simulink model "Collision_assist_system_24_08_23_new1232020"  (R2020b)
settings: Solver=FixedStepDiscrete  StartTime=0  StopTime=100  FixedStep=0.1  RelTol=1e-3
model workspace (MAT data in the model file):
  Activate_AEB = 2
  Do_nothing = 0
  M = 3
  Match_relative_speed = 1
libraries: simulink x21
settings Model: Creator=Manohar  LastModifiedBy=Manohar
settings DebuggingCC: SFUnusedDataAndEventsDiag=none  SFUnexpectedBacktrackingDiag=none  SFInvalidInputDataAccessInChartInitDiag=none  SFNoUnconditionalDefaultTransitionDiag=none  SFUndirectedBroadcastEventsDiag=none  SFOutputUsedAsStateInMooreChartDiag=none  SFMachineParentedDataDiag=none

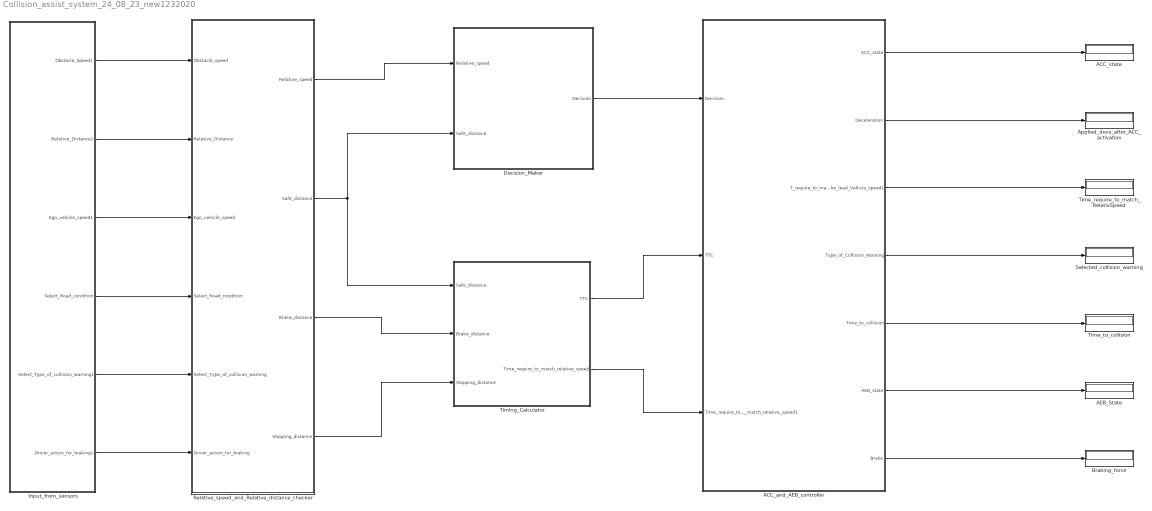
== system Collision_assist_system_24_08_23_new1232020 ==
  ACC_and_AEB_controller : Subsystem
  ACC_state : Display
  AEB_State : Display
  Applied_dece_after_ACC_activation : Display
  Braking_force : Display
  Decision_Maker : Subsystem
  Input_from_sensors : Subsystem
  Relative_speed_and_Relative_distance_checker : Subsystem
  Selected_collision_warning : Display
  Time_require_to_match_RelativSpeed : Display
  Time_to_collision : Display
  Timing_Calculator : Subsystem
  wires:
  Timing_Calculator/1(TTC) -> ACC_and_AEB_controller/2(TTC)
  ACC_and_AEB_controller/4(Type_of_Collision_Warning) -> Selected_collision_warning/1
  ACC_and_AEB_controller/5(Time_to_collision) -> Time_to_collision/1
  ACC_and_AEB_controller/6(AEB_state) -> AEB_State/1
  Relative_speed_and_Relative_distance_checker/2(Safe_distance) -> Timing_Calculator/1(Safe_distance), Decision_Maker/2(Safe_distance)
  Relative_speed_and_Relative_distance_checker/1(Relative_speed) -> Decision_Maker/1(Relative_speed)
  Relative_speed_and_Relative_distance_checker/3(Brake_distance) -> Timing_Calculator/2(Brake_distance)
  Relative_speed_and_Relative_distance_checker/4(Stopping_distance) -> Timing_Calculator/3(Stopping_distance)
  ACC_and_AEB_controller/7(Brake) -> Braking_force/1
  Decision_Maker/1(Decision) -> ACC_and_AEB_controller/1(Decision)
  Timing_Calculator/2(Time_require_to_match_relative_speed) -> ACC_and_AEB_controller/3(Time_require_to_match_relative_speed1)
  ACC_and_AEB_controller/2(Deceleration) -> Applied_dece_after_ACC_activation/1
  ACC_and_AEB_controller/1(ACC_state) -> ACC_state/1
  ACC_and_AEB_controller/3(T_require_to_match_the_lead_Vehicle_speed1) -> Time_require_to_match_RelativSpeed/1
  Input_from_sensors/1(Obstacle_Speed1) -> Relative_speed_and_Relative_distance_checker/1(Obstacle_speed)
  Input_from_sensors/2(Relative_Distance1) -> Relative_speed_and_Relative_distance_checker/2(Relative_Distance)
  Input_from_sensors/3(Ego_vehicle_speed1) -> Relative_speed_and_Relative_distance_checker/3(Ego_vehicle_speed)
  Input_from_sensors/4(Select_Road_condition) -> Relative_speed_and_Relative_distance_checker/4(Select_Road_condition)
  Input_from_sensors/5(Select_Type_of_collision_warning1) -> Relative_speed_and_Relative_distance_checker/5(Select_Type_of_collision_warning)
  Input_from_sensors/6(Driver_action_for_braking1) -> Relative_speed_and_Relative_distance_checker/6(Driver_action_for_braking)

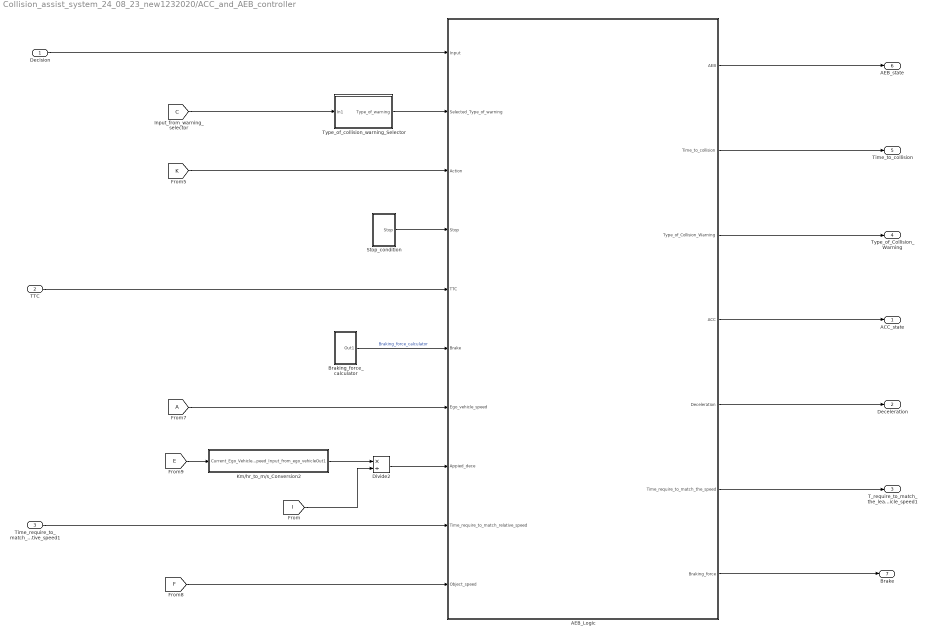
== system Collision_assist_system_24_08_23_new1232020/ACC_and_AEB_controller ==
  Decision : Inport
  TTC : Inport  Port=2
  Time_require_to_match_relative_speed1 : Inport  Port=3
  AEB_Logic : Stateflow chart  TreatAsAtomicUnit=on
      settings: PortSchema="{\"entries\":[{\"content\":{\"sides\":[{\"content\":{\"connectorIds\":[\"In5\",\"In4\",\"In3\",\"In1\",\"In2\",\"In6\",\"In7\",\"In10\",\"In8\",\"In9\"]},\"type\":\"ConnectorPlacement.EquallySpacedRectSide\",\"uuid\":\"56efa24c-13f5-4a10-8798-262846c2e7d6\"},{\"content\":{\"connectorIds\":[\"Out2\",\"Out1\",\"Out3\",\"Out5\",\"Out6\",\"Out7\",\"Out4\"],\"side\":\"RIGHT\"},\"type\":\"ConnectorPlacement.EquallySpacedRectSide\",\"uuid\":\"b772b444-91dc-49b5-b56a-5600aa3cb1ee\"},{\"content\":{\"connectorIds\":[],\"side\":\"TOP\"},\"type\":\"ConnectorPlacement.EquallySpacedRectSide\",\"uuid\":\"4494dcf3-e0bf-46dd-8a42-4684d9a2f726\"}]},\"type\":\"ConnectorPlacement.EquallySpacedConnector\",\"uuid\":\"5a6c621f-0a2a-4f9e-80e5-9478e9780666\"}],\"packageUris\":[\"http://schema.mathworks.com/mf0/Connector/R2020b\"],\"version\":\"1.0\"}"
  Braking_force_calculator : Subsystem
  Divide2 : Product  Inputs=*/
  Km/hr_to_m/s_Conversion2 : Subsystem
  Stop_condition : Subsystem
  Type_of_collision_warning_Selector : Subsystem
  ACC_state : Outport
  Deceleration : Outport  Port=2
  T_require_to_match_the_lead_Vehicle_speed1 : Outport  Port=3
  Type_of_Collision_Warning : Outport  Port=4
  Time_to_collision : Outport  Port=5
  AEB_state : Outport  Port=6
  Brake : Outport  Port=7
  wires:
  Stop_condition/1(Stop) -> AEB_Logic/1(Stop)
  [C] -> Type_of_collision_warning_Selector/1(In1)
  Type_of_collision_warning_Selector/1(Type_of_warning) -> AEB_Logic/4(Selected_Type_of_warning)
  AEB_Logic/2(AEB) -> AEB_state/1
  AEB_Logic/3(Type_of_Collision_Warning) -> Type_of_Collision_Warning/1
  TTC/1 -> AEB_Logic/2(TTC)
  [K] -> AEB_Logic/3(Action)
  AEB_Logic/4(Braking_force) -> Brake/1
  Braking_force_calculator/1(Out1) -> AEB_Logic/6(Brake)  "Braking_force_calculator"
  AEB_Logic/1(Time_to_collision) -> Time_to_collision/1
  [A] -> AEB_Logic/7(Ego_vehicle_speed)
  Divide2/1 -> AEB_Logic/10(Appied_dece)
  [E] -> Km/hr_to_m/s_Conversion2/1(Current_Ego_Vehicle_Speed_Input_from_ego_vehicle)
  Km/hr_to_m/s_Conversion2/1(Out1) -> Divide2/1
  Time_require_to_match_relative_speed1/1 -> AEB_Logic/8(Time_require_to_match_relative_speed)
  [F] -> AEB_Logic/9(Object_speed)
  AEB_Logic/6(Deceleration) -> Deceleration/1
  AEB_Logic/5(ACC) -> ACC_state/1
  AEB_Logic/7(Time_require_to_match_the_speed) -> T_require_to_match_the_lead_Vehicle_speed1/1
  Decision/1 -> AEB_Logic/5(Input)
  [I] -> Divide2/2

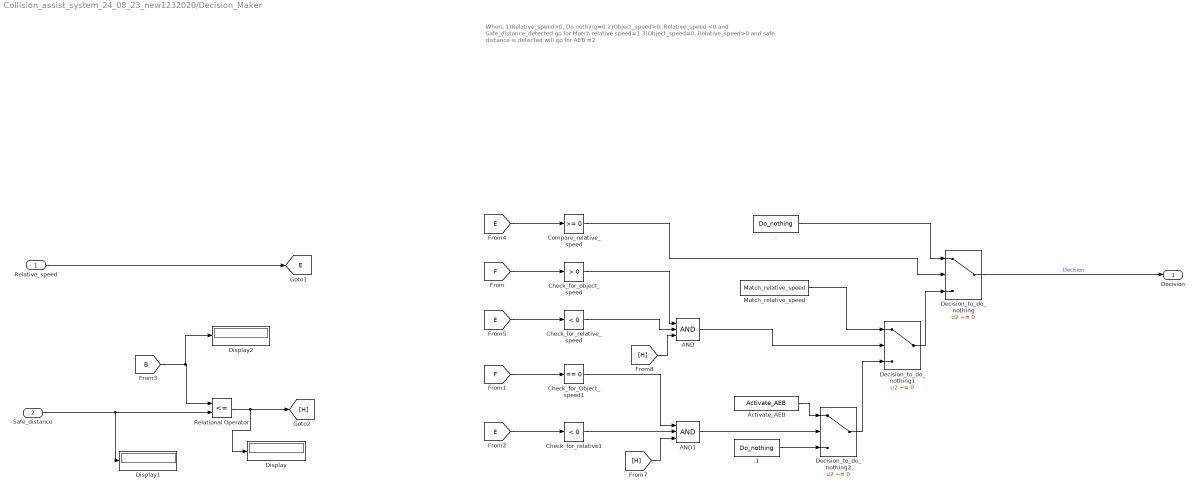
== system Collision_assist_system_24_08_23_new1232020/Decision_Maker ==
  note: When,
      | 1)Relative_speed>0, Do nothing=0
      |
      | 2)Object_speed>0, Relative_speed <0 and Safe_distance_detected go for Match relative speed=1
      |
      | 3)Object_speed=0, Relative_speed>0 and safe distance is detected will go for AEB =2
  Relative_speed : Inport
  Safe_distance : Inport  Port=2
  . : Constant  Value=Do_nothing
  .1 : Constant  Value=Do_nothing
  AND : Logic  Inputs=3  AllPortsSameDT=off  OutDataTypeStr=boolean
  AND1 : Logic  Inputs=3  AllPortsSameDT=off  OutDataTypeStr=boolean
  Activate_AEB : Constant  Value=Activate_AEB
  Check_for_Object_speed1 : simulink/Logic and Bit Operations/Compare To Constant  relop===  const=0  OutDataTypeStr=boolean
  Check_for_object_speed : simulink/Logic and Bit Operations/Compare To Constant  relop=>  const=0  OutDataTypeStr=boolean
  Check_for_relative1 : simulink/Logic and Bit Operations/Compare To Constant  relop=<  const=0  OutDataTypeStr=boolean
  Check_for_relative_speed : simulink/Logic and Bit Operations/Compare To Constant  relop=<  const=0  OutDataTypeStr=boolean
  Compare_relative_speed : simulink/Logic and Bit Operations/Compare To Constant  relop=>=  const=0  OutDataTypeStr=boolean
  Decision_to_do_nothing : Switch  Criteria=u2 ~= 0
  Decision_to_do_nothing1 : Switch  Criteria=u2 ~= 0
  Decision_to_do_nothing2 : Switch  Criteria=u2 ~= 0
  Display : Display
  Display1 : Display
  Display2 : Display
  Match_relative_speed : Constant  Value=Match_relative_speed
  Relational Operator : RelationalOperator  Operator=<=  OutDataTypeStr=boolean  RndMeth=Simplest
  Decision : Outport
  tag scope: E=global
  wires:
  [B] -> Display2/1, Relational Operator/1
  Decision_to_do_nothing1/1 -> Decision_to_do_nothing/3
  Compare_relative_speed/1 -> Decision_to_do_nothing/2
  Decision_to_do_nothing/1 -> Decision/1  "Decision"
  Match_relative_speed/1 -> Decision_to_do_nothing1/1
  ./1 -> Decision_to_do_nothing/1
  Check_for_object_speed/1 -> AND/1
  Check_for_relative_speed/1 -> AND/2
  AND/1 -> Decision_to_do_nothing1/2
  Relative_speed/1 -> [E]
  Decision_to_do_nothing2/1 -> Decision_to_do_nothing1/3
  Activate_AEB/1 -> Decision_to_do_nothing2/1
  AND1/1 -> Decision_to_do_nothing2/2
  [F] -> Check_for_object_speed/1
  [F] -> Check_for_Object_speed1/1
  [E] -> Check_for_relative1/1
  Check_for_relative1/1 -> AND1/2
  Check_for_Object_speed1/1 -> AND1/1
  Safe_distance/1 -> Display1/1, Relational Operator/2
  [E] -> Compare_relative_speed/1
  [E] -> Check_for_relative_speed/1
  Relational Operator/1 -> Display/1, [H]
  [H] -> AND1/3
  [H] -> AND/3
  .1/1 -> Decision_to_do_nothing2/3

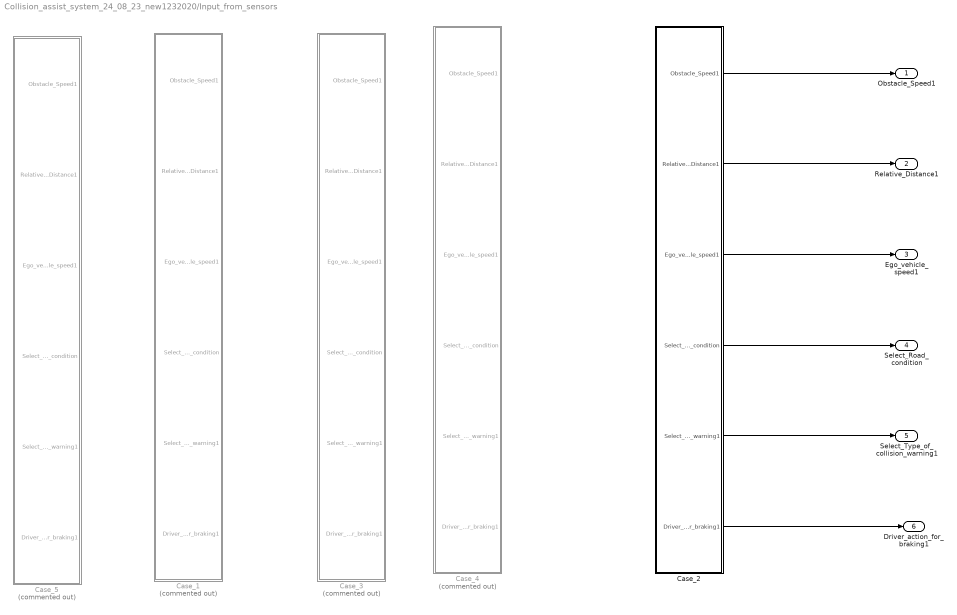
== system Collision_assist_system_24_08_23_new1232020/Input_from_sensors ==
  Case_1 : Subsystem  Commented=on
  Case_2 : Subsystem
  Case_3 : Subsystem  Commented=on
  Case_4 : Subsystem  Commented=on
  Case_5 : Subsystem  Commented=on
  Obstacle_Speed1 : Outport
  Relative_Distance1 : Outport  Port=2
  Ego_vehicle_speed1 : Outport  Port=3
  Select_Road_condition : Outport  Port=4
  Select_Type_of_collision_warning1 : Outport  Port=5
  Driver_action_for_braking1 : Outport  Port=6
  wires:
  Case_2/1(Obstacle_Speed1) -> Obstacle_Speed1/1
  Case_2/2(Relative_Distance1) -> Relative_Distance1/1
  Case_2/3(Ego_vehicle_speed1) -> Ego_vehicle_speed1/1
  Case_2/4(Select_Road_condition) -> Select_Road_condition/1
  Case_2/5(Select_Type_of_collision_warning1) -> Select_Type_of_collision_warning1/1
  Case_2/6(Driver_action_for_braking1) -> Driver_action_for_braking1/1

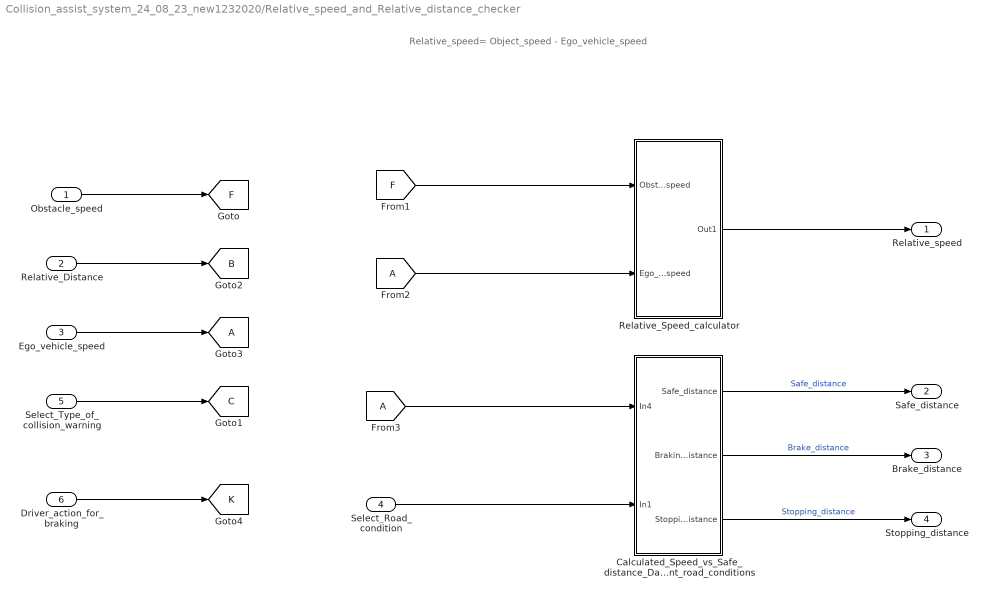
== system Collision_assist_system_24_08_23_new1232020/Relative_speed_and_Relative_distance_checker ==
  note: Relative_speed= Object_speed - Ego_vehicle_speed
  Obstacle_speed : Inport
  Relative_Distance : Inport  Port=2
  Ego_vehicle_speed : Inport  Port=3
  Select_Road_condition : Inport  Port=4
  Select_Type_of_collision_warning : Inport  Port=5
  Driver_action_for_braking : Inport  Port=6
  Calculated_Speed_vs_Safe_distance_Data_based_on_different_road_conditions : Subsystem
  Relative_Speed_calculator : Subsystem
  Relative_speed : Outport
  Safe_distance : Outport  Port=2
  Brake_distance : Outport  Port=3
  Stopping_distance : Outport  Port=4
  tag scope: A=global, B=global, C=global, F=global, K=global
  wires:
  Ego_vehicle_speed/1 -> [A]
  Calculated_Speed_vs_Safe_distance_Data_based_on_different_road_conditions/1(Safe_distance) -> Safe_distance/1  "Safe_distance"
  Relative_Distance/1 -> [B]
  Select_Road_condition/1 -> Calculated_Speed_vs_Safe_distance_Data_based_on_different_road_conditions/2(In1)
  Select_Type_of_collision_warning/1 -> [C]
  Relative_Speed_calculator/1(Out1) -> Relative_speed/1
  Calculated_Speed_vs_Safe_distance_Data_based_on_different_road_conditions/2(Braking_distance) -> Brake_distance/1  "Brake_distance"
  Calculated_Speed_vs_Safe_distance_Data_based_on_different_road_conditions/3(Stopping_distance) -> Stopping_distance/1  "Stopping_distance"
  Obstacle_speed/1 -> [F]
  [F] -> Relative_Speed_calculator/1(Obstacle_speed)
  [A] -> Relative_Speed_calculator/2(Ego_vehicle_speed)
  [A] -> Calculated_Speed_vs_Safe_distance_Data_based_on_different_road_conditions/1(In4)
  Driver_action_for_braking/1 -> [K]

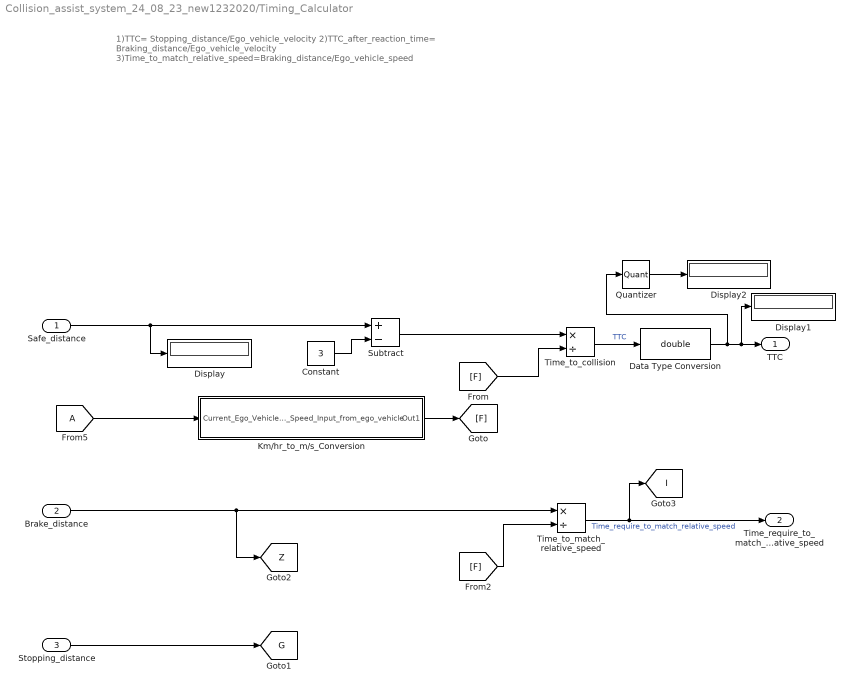
== system Collision_assist_system_24_08_23_new1232020/Timing_Calculator ==
  note: 1)TTC= Stopping_distance/Ego_vehicle_velocity
      |
      | 2)TTC_after_reaction_time= Braking_distance/Ego_vehicle_velocity
      |
      | 3)Time_to_match_relative_speed=Braking_distance/Ego_vehicle_speed
  Safe_distance : Inport
  Brake_distance : Inport  Port=2
  Stopping_distance : Inport  Port=3
  Constant : Constant  Value=3
  Data Type Conversion : DataTypeConversion  OutDataTypeStr=double
  Display : Display
  Display1 : Display
  Display2 : Display
  Km/hr_to_m/s_Conversion : Subsystem
  Quantizer : Quantizer  QuantizationInterval=0.4
  Subtract : Sum  Inputs=+-
  Time_to_collision : Product  Inputs=*/  RndMeth=Zero
  Time_to_match_relative_speed : Product  Inputs=*/
  TTC : Outport
  Time_require_to_match_relative_speed : Outport  Port=2
  tag scope: G=global, I=global, Z=global
  wires:
  Safe_distance/1 -> Display/1, Subtract/1
  Constant/1 -> Subtract/2
  Subtract/1 -> Time_to_collision/1
  Brake_distance/1 -> [Z], Time_to_match_relative_speed/1
  Time_to_match_relative_speed/1 -> [I], Time_require_to_match_relative_speed/1  "Time_require_to_match_relative_speed"
  Km/hr_to_m/s_Conversion/1(Out1) -> [F]
  [F] -> Time_to_collision/2
  [F] -> Time_to_match_relative_speed/2
  Stopping_distance/1 -> [G]
  [A] -> Km/hr_to_m/s_Conversion/1(Current_Ego_Vehicle_Speed_Input_from_ego_vehicle)
  Time_to_collision/1 -> Data Type Conversion/1  "TTC"
  Data Type Conversion/1 -> Quantizer/1, Display1/1, TTC/1
  Quantizer/1 -> Display2/1

== system Collision_assist_system_24_08_23_new1232020/ACC_and_AEB_controller/Braking_force_calculator ==
  Constant : Constant  Value=0.5
  Constant1 : Constant  Value=1500
  Display : Display
  Divide1 : Product  Inputs=*/
  Km/hr_to_m/s_Conversion : Subsystem
  Product : Product  Inputs=3
  Square : Math  Operator=square  SaturateOnIntegerOverflow=on
  Out1 : Outport
  wires:
  Constant/1 -> Product/1
  Product/1 -> Divide1/1
  Constant1/1 -> Product/2
  Divide1/1 -> Display/1, Out1/1
  [Z] -> Divide1/2
  [A] -> Km/hr_to_m/s_Conversion/1(Current_Ego_Vehicle_Speed_Input_from_ego_vehicle)
  Square/1 -> Product/3
  Km/hr_to_m/s_Conversion/1(Out1) -> Square/1

== system Collision_assist_system_24_08_23_new1232020/ACC_and_AEB_controller/Km//hr_to_m//s_Conversion2 ==
  note: 1(km/hr)=1/3.6(m/s)
  Current_Ego_Vehicle_Speed_Input_from_ego_vehicle : Inport
  Constant : Constant  Value=3.6
  Divide : Product  Inputs=*/
  Out1 : Outport
  wires:
  Current_Ego_Vehicle_Speed_Input_from_ego_vehicle/1 -> Divide/1
  Constant/1 -> Divide/2
  Divide/1 -> Out1/1

== system Collision_assist_system_24_08_23_new1232020/ACC_and_AEB_controller/Stop_condition ==
  Compare To Constant : simulink/Logic and Bit Operations/Compare To Constant  relop===  const=0  OutDataTypeStr=boolean
  Constant : Constant
  Constant1 : Constant  Value=0
  Switch : Switch  Criteria=u2 > Threshold
  Stop : Outport
  wires:
  Switch/1 -> Stop/1
  [A] -> Compare To Constant/1
  Compare To Constant/1 -> Switch/2
  Constant/1 -> Switch/1
  Constant1/1 -> Switch/3

== system Collision_assist_system_24_08_23_new1232020/ACC_and_AEB_controller/Type_of_collision_warning_Selector ==
  In1 : Inport
  Audiable : Constant  Value=2
  Haptic : Constant  Value=3
  Multiport Switch : MultiPortSwitch
  Visual : Constant
  Type_of_warning : Outport
  wires:
  Multiport Switch/1 -> Type_of_warning/1
  In1/1 -> Multiport Switch/1
  Visual/1 -> Multiport Switch/2
  Audiable/1 -> Multiport Switch/3
  Haptic/1 -> Multiport Switch/4

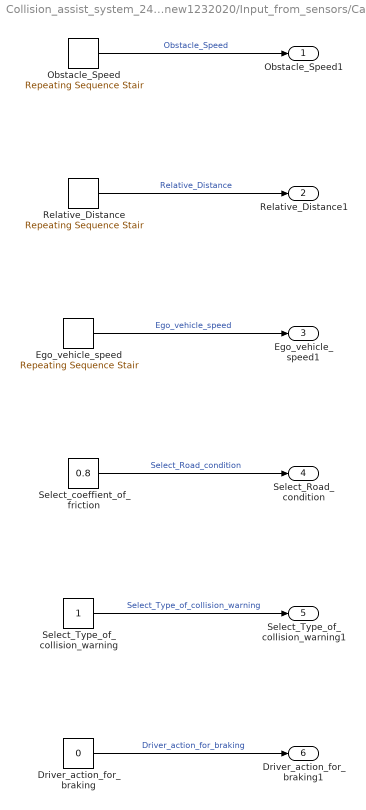
== system Collision_assist_system_24_08_23_new1232020/Input_from_sensors/Case_1 ==
  Driver_action_for_braking : Constant  Value=0
  Ego_vehicle_speed : simulink/Sources/Repeating Sequence Stair  OutValues=[50 50 50 50 50 40 35 30 25 20 15 10 0 0 ].'  tsamp=-1  OutMin=[]  OutMax=[]  OutDataTypeStr=double  OutputDataTypeScalingMode=double  OutDataType=fixdt(0,8)  ConRadixGroup=Best Precision: Vector-wise  OutScaling=2^-12
  Obstacle_Speed : simulink/Sources/Repeating Sequence Stair  OutValues="[0 0 0 0 0 0 0 0 0 0 0 0 0 0  ]"  tsamp=-1  OutMin=[]  OutMax=[]  OutDataTypeStr=double  OutputDataTypeScalingMode=double  OutDataType=fixdt(0,8)  ConRadixGroup=Best Precision: Vector-wise  OutScaling=2^-12
  Relative_Distance : simulink/Sources/Repeating Sequence Stair  OutValues=[20.84 ]  tsamp=-1  OutMin=[]  OutMax=[]  OutDataTypeStr=double  OutputDataTypeScalingMode=double  OutDataType=fixdt(0,8)  ConRadixGroup=Best Precision: Vector-wise  OutScaling=2^-12
  Select_Type_of_collision_warning : Constant
  Select_coeffient_of_friction : Constant  Value=0.8
  Obstacle_Speed1 : Outport
  Relative_Distance1 : Outport  Port=2
  Ego_vehicle_speed1 : Outport  Port=3
  Select_Road_condition : Outport  Port=4
  Select_Type_of_collision_warning1 : Outport  Port=5
  Driver_action_for_braking1 : Outport  Port=6
  wires:
  Select_coeffient_of_friction/1 -> Select_Road_condition/1  "Select_Road_condition"
  Ego_vehicle_speed/1 -> Ego_vehicle_speed1/1  "Ego_vehicle_speed"
  Relative_Distance/1 -> Relative_Distance1/1  "Relative_Distance"
  Select_Type_of_collision_warning/1 -> Select_Type_of_collision_warning1/1  "Select_Type_of_collision_warning"
  Obstacle_Speed/1 -> Obstacle_Speed1/1  "Obstacle_Speed"
  Driver_action_for_braking/1 -> Driver_action_for_braking1/1  "Driver_action_for_braking"

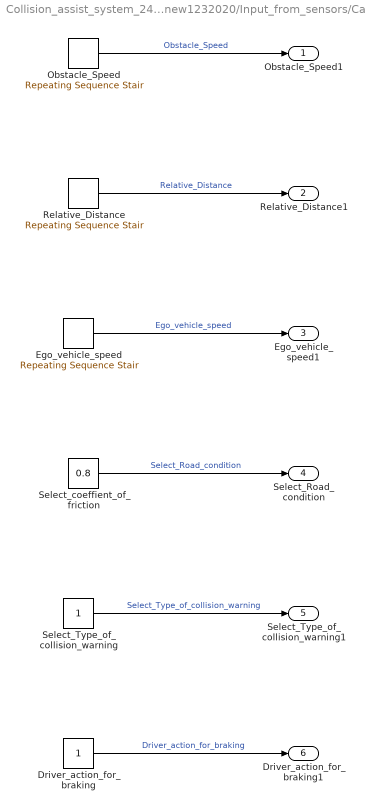
== system Collision_assist_system_24_08_23_new1232020/Input_from_sensors/Case_2 ==
  Driver_action_for_braking : Constant
  Ego_vehicle_speed : simulink/Sources/Repeating Sequence Stair  OutValues=[50 50 50 50 50 40 35 30 25 20 15 10 0 0 ].'  tsamp=-1  OutMin=[]  OutMax=[]  OutDataTypeStr=double  OutputDataTypeScalingMode=double  OutDataType=fixdt(0,8)  ConRadixGroup=Best Precision: Vector-wise  OutScaling=2^-12
  Obstacle_Speed : simulink/Sources/Repeating Sequence Stair  OutValues="[0  ]"  tsamp=-1  OutMin=[]  OutMax=[]  OutDataTypeStr=double  OutputDataTypeScalingMode=double  OutDataType=fixdt(0,8)  ConRadixGroup=Best Precision: Vector-wise  OutScaling=2^-12
  Relative_Distance : simulink/Sources/Repeating Sequence Stair  OutValues=[20.84 ]  tsamp=-1  OutMin=[]  OutMax=[]  OutDataTypeStr=double  OutputDataTypeScalingMode=double  OutDataType=fixdt(0,8)  ConRadixGroup=Best Precision: Vector-wise  OutScaling=2^-12
  Select_Type_of_collision_warning : Constant
  Select_coeffient_of_friction : Constant  Value=0.8
  Obstacle_Speed1 : Outport
  Relative_Distance1 : Outport  Port=2
  Ego_vehicle_speed1 : Outport  Port=3
  Select_Road_condition : Outport  Port=4
  Select_Type_of_collision_warning1 : Outport  Port=5
  Driver_action_for_braking1 : Outport  Port=6
  wires:
  Driver_action_for_braking/1 -> Driver_action_for_braking1/1  "Driver_action_for_braking"
  Obstacle_Speed/1 -> Obstacle_Speed1/1  "Obstacle_Speed"
  Select_Type_of_collision_warning/1 -> Select_Type_of_collision_warning1/1  "Select_Type_of_collision_warning"
  Relative_Distance/1 -> Relative_Distance1/1  "Relative_Distance"
  Ego_vehicle_speed/1 -> Ego_vehicle_speed1/1  "Ego_vehicle_speed"
  Select_coeffient_of_friction/1 -> Select_Road_condition/1  "Select_Road_condition"

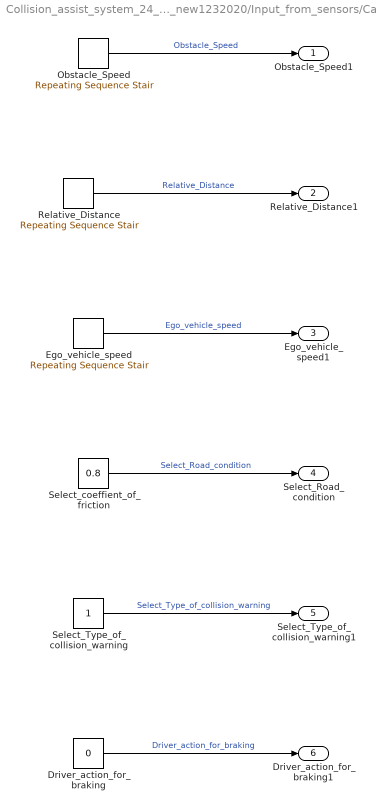
== system Collision_assist_system_24_08_23_new1232020/Input_from_sensors/Case_3 ==
  Driver_action_for_braking : Constant  Value=0
  Ego_vehicle_speed : simulink/Sources/Repeating Sequence Stair  OutValues=[50 50 50 50 50 50 50 45 40 35 30 25 22 20 20 20 ].'  tsamp=-1  OutMin=[]  OutMax=[]  OutDataTypeStr=double  OutputDataTypeScalingMode=double  OutDataType=fixdt(0,8)  ConRadixGroup=Best Precision: Vector-wise  OutScaling=2^-12
  Obstacle_Speed : simulink/Sources/Repeating Sequence Stair  OutValues=[20 ]  tsamp=-1  OutMin=[]  OutMax=[]  OutDataTypeStr=double  OutputDataTypeScalingMode=double  OutDataType=fixdt(0,8)  ConRadixGroup=Best Precision: Vector-wise  OutScaling=2^-12
  Relative_Distance : simulink/Sources/Repeating Sequence Stair  OutValues=[20.84 ]  tsamp=-1  OutMin=[]  OutMax=[]  OutDataTypeStr=double  OutputDataTypeScalingMode=double  OutDataType=fixdt(0,8)  ConRadixGroup=Best Precision: Vector-wise  OutScaling=2^-12
  Select_Type_of_collision_warning : Constant
  Select_coeffient_of_friction : Constant  Value=0.8
  Obstacle_Speed1 : Outport
  Relative_Distance1 : Outport  Port=2
  Ego_vehicle_speed1 : Outport  Port=3
  Select_Road_condition : Outport  Port=4
  Select_Type_of_collision_warning1 : Outport  Port=5
  Driver_action_for_braking1 : Outport  Port=6
  wires:
  Select_coeffient_of_friction/1 -> Select_Road_condition/1  "Select_Road_condition"
  Ego_vehicle_speed/1 -> Ego_vehicle_speed1/1  "Ego_vehicle_speed"
  Relative_Distance/1 -> Relative_Distance1/1  "Relative_Distance"
  Select_Type_of_collision_warning/1 -> Select_Type_of_collision_warning1/1  "Select_Type_of_collision_warning"
  Obstacle_Speed/1 -> Obstacle_Speed1/1  "Obstacle_Speed"
  Driver_action_for_braking/1 -> Driver_action_for_braking1/1  "Driver_action_for_braking"

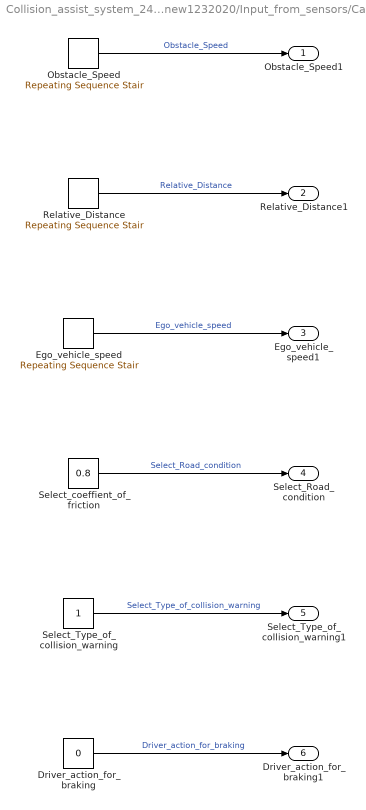
== system Collision_assist_system_24_08_23_new1232020/Input_from_sensors/Case_4 ==
  Driver_action_for_braking : Constant  Value=0
  Ego_vehicle_speed : simulink/Sources/Repeating Sequence Stair  OutValues=[50 ].'  tsamp=-1  OutMin=[]  OutMax=[]  OutDataTypeStr=double  OutputDataTypeScalingMode=double  OutDataType=fixdt(0,8)  ConRadixGroup=Best Precision: Vector-wise  OutScaling=2^-12
  Obstacle_Speed : simulink/Sources/Repeating Sequence Stair  OutValues=60  tsamp=-1  OutMin=[]  OutMax=[]  OutDataTypeStr=double  OutputDataTypeScalingMode=double  OutDataType=fixdt(0,8)  ConRadixGroup=Best Precision: Vector-wise  OutScaling=2^-12
  Relative_Distance : simulink/Sources/Repeating Sequence Stair  OutValues=[20.84 ]  tsamp=-1  OutMin=[]  OutMax=[]  OutDataTypeStr=double  OutputDataTypeScalingMode=double  OutDataType=fixdt(0,8)  ConRadixGroup=Best Precision: Vector-wise  OutScaling=2^-12
  Select_Type_of_collision_warning : Constant
  Select_coeffient_of_friction : Constant  Value=0.8
  Obstacle_Speed1 : Outport
  Relative_Distance1 : Outport  Port=2
  Ego_vehicle_speed1 : Outport  Port=3
  Select_Road_condition : Outport  Port=4
  Select_Type_of_collision_warning1 : Outport  Port=5
  Driver_action_for_braking1 : Outport  Port=6
  wires:
  Driver_action_for_braking/1 -> Driver_action_for_braking1/1  "Driver_action_for_braking"
  Obstacle_Speed/1 -> Obstacle_Speed1/1  "Obstacle_Speed"
  Select_Type_of_collision_warning/1 -> Select_Type_of_collision_warning1/1  "Select_Type_of_collision_warning"
  Relative_Distance/1 -> Relative_Distance1/1  "Relative_Distance"
  Ego_vehicle_speed/1 -> Ego_vehicle_speed1/1  "Ego_vehicle_speed"
  Select_coeffient_of_friction/1 -> Select_Road_condition/1  "Select_Road_condition"

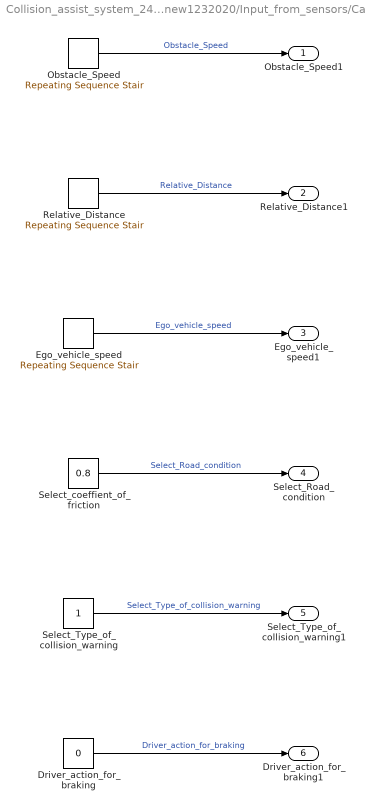
== system Collision_assist_system_24_08_23_new1232020/Input_from_sensors/Case_5 ==
  Driver_action_for_braking : Constant  Value=0
  Ego_vehicle_speed : simulink/Sources/Repeating Sequence Stair  OutValues=[30 30 30 30 ].'  tsamp=-1  OutMin=[]  OutMax=[]  OutDataTypeStr=double  OutputDataTypeScalingMode=double  OutDataType=fixdt(0,8)  ConRadixGroup=Best Precision: Vector-wise  OutScaling=2^-12
  Obstacle_Speed : simulink/Sources/Repeating Sequence Stair  OutValues="[0 20 30 40 50 60 60 60 60 70 80 90 100 120  ]"  tsamp=-1  OutMin=[]  OutMax=[]  OutDataTypeStr=double  OutputDataTypeScalingMode=double  OutDataType=fixdt(0,8)  ConRadixGroup=Best Precision: Vector-wise  OutScaling=2^-12
  Relative_Distance : simulink/Sources/Repeating Sequence Stair  OutValues=[10.75 ]  tsamp=-1  OutMin=[]  OutMax=[]  OutDataTypeStr=double  OutputDataTypeScalingMode=double  OutDataType=fixdt(0,8)  ConRadixGroup=Best Precision: Vector-wise  OutScaling=2^-12
  Select_Type_of_collision_warning : Constant
  Select_coeffient_of_friction : Constant  Value=0.8
  Obstacle_Speed1 : Outport
  Relative_Distance1 : Outport  Port=2
  Ego_vehicle_speed1 : Outport  Port=3
  Select_Road_condition : Outport  Port=4
  Select_Type_of_collision_warning1 : Outport  Port=5
  Driver_action_for_braking1 : Outport  Port=6
  wires:
  Select_coeffient_of_friction/1 -> Select_Road_condition/1  "Select_Road_condition"
  Ego_vehicle_speed/1 -> Ego_vehicle_speed1/1  "Ego_vehicle_speed"
  Relative_Distance/1 -> Relative_Distance1/1  "Relative_Distance"
  Select_Type_of_collision_warning/1 -> Select_Type_of_collision_warning1/1  "Select_Type_of_collision_warning"
  Obstacle_Speed/1 -> Obstacle_Speed1/1  "Obstacle_Speed"
  Driver_action_for_braking/1 -> Driver_action_for_braking1/1  "Driver_action_for_braking"

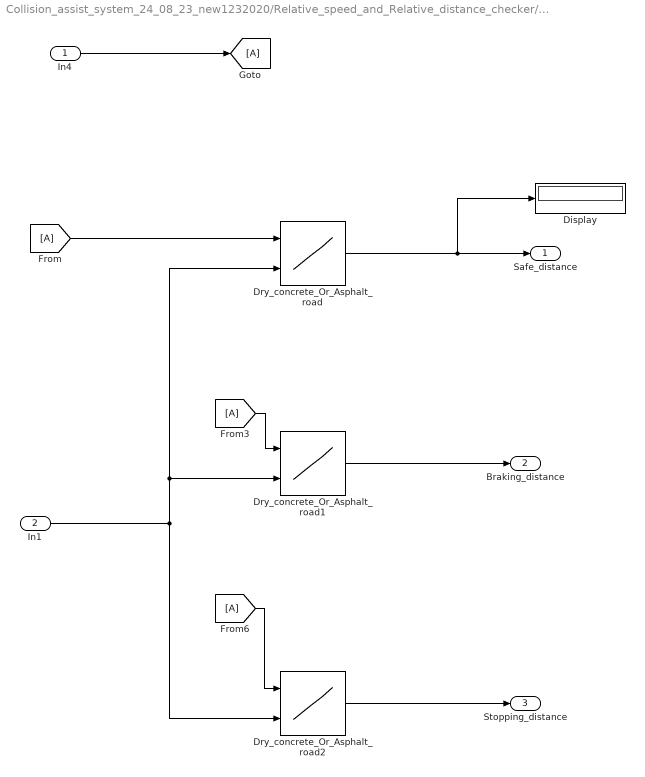
== system Collision_assist_system_24_08_23_new1232020/Relative_speed_and_Relative_distance_checker/Calculated_Speed_vs_Safe_distance_Data_based_on_different_road_conditions ==
  In4 : Inport
  In1 : Inport  Port=2
  Display : Display
  Dry_concrete_Or_Asphalt_road : Lookup_n-D  BreakpointsForDimension1=[30:10:120]  BreakpointsForDimension2=[0.2,0.5,0.8]  BreakpointsForDimension3=[5, 7]  Table=[24.03 38.91 57.71 80.46 107.1 137.7 172.3 210.7 253.2 299.5; 13.41 20.03 28.22 37.98 49.32 62.23 76.71 92.77 110.4 129.6; 10.75 15.3 20.84 27.36 34.84 43.33 52.81 63.27 74.72 87.1 ].'  InternalRulePriority=Speed  RndMeth=Simplest  InputSameDT=on
      settings: InputPortMap=u0,u1
  Dry_concrete_Or_Asphalt_road1 : Lookup_n-D  BreakpointsForDimension1=[30:10:120]  BreakpointsForDimension2=[0.2,0.5,0.8]  BreakpointsForDimension3=[5, 7]  Table=[17.7 31.46 49.16 70.79 96.35 125.8 159.3 196.6 237.9 283.2; 7.07 12.58 19.66 28.32 38.54 50.34 63.71 78.65 95.17 113.3; 4.42 7.86 12.29 17.7 24.07 31.45 39.81 49.16 59.5 70.77].'  InternalRulePriority=Speed  RndMeth=Simplest  InputSameDT=on
      settings: InputPortMap=u0,u1
  Dry_concrete_Or_Asphalt_road2 : Lookup_n-D  BreakpointsForDimension1=[30:10:120]  BreakpointsForDimension2=[0.2,0.5,0.8]  BreakpointsForDimension3=[5, 7]  Table=[21.03 35.91 54.71 77.46 104.1 134.7 169.3 207.7 250.2 296.5; 10.41 17.03 25.22 34.98 46.32 59.23 73.71 89.77 107.4 126.6; 7.75 12.3 17.84 24.36 31.84 40.33 49.81 60.27 71.72 84.1].'  InternalRulePriority=Speed  RndMeth=Simplest  InputSameDT=on
      settings: InputPortMap=u0,u1
  Safe_distance : Outport
  Braking_distance : Outport  Port=2
  Stopping_distance : Outport  Port=3
  wires:
  In4/1 -> [A]
  [A] -> Dry_concrete_Or_Asphalt_road/1
  Dry_concrete_Or_Asphalt_road/1 -> Display/1, Safe_distance/1
  In1/1 -> Dry_concrete_Or_Asphalt_road/2, Dry_concrete_Or_Asphalt_road1/2, Dry_concrete_Or_Asphalt_road2/2
  Dry_concrete_Or_Asphalt_road1/1 -> Braking_distance/1
  [A] -> Dry_concrete_Or_Asphalt_road1/1
  [A] -> Dry_concrete_Or_Asphalt_road2/1
  Dry_concrete_Or_Asphalt_road2/1 -> Stopping_distance/1

== system Collision_assist_system_24_08_23_new1232020/Relative_speed_and_Relative_distance_checker/Relative_Speed_calculator ==
  Obstacle_speed : Inport
  Ego_vehicle_speed : Inport  Port=2
  Subtract : Sum  Inputs=+-
  Out1 : Outport
  wires:
  Subtract/1 -> Out1/1  "Relative_speed"
  Obstacle_speed/1 -> Subtract/1
  Ego_vehicle_speed/1 -> Subtract/2

== system Collision_assist_system_24_08_23_new1232020/Timing_Calculator/Km//hr_to_m//s_Conversion ==
  note: 1(km/hr)=1/3.6(m/s)
  Current_Ego_Vehicle_Speed_Input_from_ego_vehicle : Inport
  Constant : Constant  Value=3.6
  Divide : Product  Inputs=*/
  Out1 : Outport
  wires:
  Current_Ego_Vehicle_Speed_Input_from_ego_vehicle/1 -> Divide/1
  Constant/1 -> Divide/2
  Divide/1 -> Out1/1

== system Collision_assist_system_24_08_23_new1232020/ACC_and_AEB_controller/Braking_force_calculator/Km//hr_to_m//s_Conversion ==
  note: 1(km/hr)=1/3.6(m/s)
  Current_Ego_Vehicle_Speed_Input_from_ego_vehicle : Inport
  Constant : Constant  Value=3.6
  Divide : Product  Inputs=*/
  Out1 : Outport
  wires:
  Current_Ego_Vehicle_Speed_Input_from_ego_vehicle/1 -> Divide/1
  Constant/1 -> Divide/2
  Divide/1 -> Out1/1

== stateflow chart Collision_assist_system_24_08_23_new1232020/ACC_and_AEB_controller/AEB_Logic ==
  state Collision_warning_generator [parallel]
    settings: executionOrder=3
    state Collision_warning_generator_Initial_state
      Type_of_Collision_Warning=0;
    state Collision_warning_generator_state3
      Type_of_Collision_Warning=Selected_Type_of_warning;
    state Collision_warning_state
      Type_of_Collision_Warning=Selected_Type_of_warning;
    state Collision_warning_generator_state1
      Type_of_Collision_Warning=Selected_Type_of_warning;
    state Collision_warning_generator_state2
      Type_of_Collision_Warning=Selected_Type_of_warning;
    state Collision_warning_state4
      Type_of_Collision_Warning=Selected_Type_of_warning;
    (default) -> Collision_warning_generator_Initial_state
    Collision_warning_state -> Collision_warning_generator_state1 [order 1] : [Object_speed<Ego_vehicle_speed]
    Collision_warning_generator_Initial_state -> Collision_warning_state : [(Input==1)||(Input==2)]
    Collision_warning_generator_state2 -> Collision_warning_generator_state3 [order 1] : [Object_speed<Ego_vehicle_speed]
    Collision_warning_generator_state1 -> Collision_warning_generator_state2 [order 1] : [Object_speed<Ego_vehicle_speed]
    (junction 270) -> Collision_warning_generator_Initial_state [order 2] : [[(Object_speed>Ego_vehicle_speed)||(Object_speed==Ego_vehicle_speed)||(Ego_vehicle_speed==0)]]
    Collision_warning_generator_state2 -> Collision_warning_generator_Initial_state [order 2] : [[(Object_speed>Ego_vehicle_speed)||(Object_speed==Ego_vehicle_speed)||(Ego_vehicle_speed==0)]]
    Collision_warning_generator_state1 -> Collision_warning_generator_Initial_state [order 2] : [[(Object_speed>Ego_vehicle_speed)||(Object_speed==Ego_vehicle_speed)||(Ego_vehicle_speed==0)]]
    Collision_warning_state -> Collision_warning_generator_Initial_state [order 2] : [[(Object_speed>Ego_vehicle_speed)||(Object_speed==Ego_vehicle_speed)||(Ego_vehicle_speed==0)]]
    (junction 271) -> Collision_warning_generator_Initial_state
    Collision_warning_generator_state3 -> (junction 270)
    (junction 270) -> Collision_warning_state4 [order 1] : [Object_speed<Ego_vehicle_speed]
    Collision_warning_state4 -> (junction 272) : [[(Object_speed>Ego_vehicle_speed)||(Object_speed==Ego_vehicle_speed)||(Ego_vehicle_speed==0)]]
    (junction 272) -> (junction 271)
  state ACC [parallel]
    settings: executionOrder=1
    state ACC_initial_state
      Deceleration=0;
      ACC=0;
      Time_require_to_match_the_speed==0;
    state ACC_non_active_state3
      Deceleration=0;
      ACC=0;
      Time_require_to_match_the_speed=0;
    state ACC_non_active_state
      Deceleration=0;
      ACC=0;
      Time_require_to_match_the_speed=0;
    state ACC_non_active_state1
      Deceleration=0;
      ACC=0;
      Time_require_to_match_the_speed=0;
    state ACC_non_active_state2
      Deceleration=0;
      ACC=0;
      Time_require_to_match_the_speed=0;
    state ACC_active_state
      en:
      Deceleration=Appied_dece;
      ACC=1;
      Time_require_to_match_the_speed=Time_require_to_match_relative_speed;
      du:
      Time_require_to_match_the_speed= Time_require_to_match_the_speed-0.1;
      ex:
      Time_require_to_match_the_speed=0;Deceleration=0;
    (default) -> ACC_initial_state
    ACC_non_active_state -> ACC_non_active_state1 [order 1] : [Object_speed<Ego_vehicle_speed]
    ACC_initial_state -> ACC_non_active_state : [Input==1]
    ACC_non_active_state2 -> ACC_non_active_state3 [order 1] : [Object_speed<Ego_vehicle_speed]
    ACC_non_active_state1 -> ACC_non_active_state2 [order 1] : [Object_speed<Ego_vehicle_speed]
    (junction 202) -> ACC_initial_state [order 2] : [[(Object_speed>Ego_vehicle_speed)||(Object_speed==Ego_vehicle_speed)||(Ego_vehicle_speed==0)]]
    ACC_non_active_state2 -> ACC_initial_state [order 2] : [[(Object_speed>Ego_vehicle_speed)||(Object_speed==Ego_vehicle_speed)||(Ego_vehicle_speed==0)]]
    ACC_non_active_state1 -> ACC_initial_state [order 2] : [[(Object_speed>Ego_vehicle_speed)||(Object_speed==Ego_vehicle_speed)||(Ego_vehicle_speed==0)]]
    ACC_non_active_state -> ACC_initial_state [order 2] : [[(Object_speed>Ego_vehicle_speed)||(Object_speed==Ego_vehicle_speed)||(Ego_vehicle_speed==0)]]
    (junction 166) -> ACC_initial_state
    ACC_non_active_state3 -> (junction 202)
    (junction 202) -> ACC_active_state [order 1] : [Object_speed<Ego_vehicle_speed]
    ACC_active_state -> (junction 169) : [[(Object_speed>Ego_vehicle_speed)||(Object_speed==Ego_vehicle_speed)||(Ego_vehicle_speed==0)]]
    (junction 169) -> (junction 166)
  state AEB [parallel]
    settings: executionOrder=2
    state AEB_initial_state
      AEB=0;
      Time_to_collision=0;
    state Warning_state1
      AEB=0;
      Time_to_collision=Time_to_collision-0.1;
      ex:Time_to_collision=Time_to_collision;
    state Warning_state2
      en:
      AEB=0;
      Time_to_collision=Time_to_collision-0.1;
      ex:Time_to_collision=Time_to_collision;
    state Warning_state3
      en:
      AEB=0;
      Time_to_collision=Time_to_collision-0.1;
      du:Time_to_collision=Time_to_collision-0.1;
      ex:Time_to_collision=Time_to_collision;
    state Warning_state
      en:
      AEB=0;
      Time_to_collision=TTC-0.1;
      ex:Time_to_collision=Time_to_collision
    state AEB_activation_state
      en:
      AEB=1;
      Time_to_collision=Time_to_collision-0.1;
      Braking_force=Brake;
      du:Time_to_collision=Time_to_collision-0.1;
      ex:Braking_force=0;
    (default) -> AEB_initial_state
    Warning_state1 -> Warning_state2 [order 1] : [Object_speed<Ego_vehicle_speed]
    Warning_state2 -> Warning_state3 [order 1] : [Object_speed<Ego_vehicle_speed]
    AEB_initial_state -> Warning_state : [Input==2]
    Warning_state -> Warning_state1 [order 1] : [Object_speed<Ego_vehicle_speed]
    Warning_state3 -> AEB_initial_state [order 2] : [(Object_speed>Ego_vehicle_speed)||(Object_speed==Ego_vehicle_speed)||(Ego_vehicle_speed==0)]
    Warning_state2 -> AEB_initial_state [order 2] : [(Object_speed>Ego_vehicle_speed)||(Object_speed==Ego_vehicle_speed)||(Ego_vehicle_speed==0)]
    Warning_state1 -> AEB_initial_state [order 2] : [[(Object_speed>Ego_vehicle_speed)||(Object_speed==Ego_vehicle_speed)||(Ego_vehicle_speed==0)]]
    Warning_state3 -> AEB_activation_state [order 1] : [(Action==0)&&(Input==2)]
    Warning_state -> AEB_initial_state [order 2] : [[(Object_speed>Ego_vehicle_speed)||(Object_speed==Ego_vehicle_speed)||(Ego_vehicle_speed==0)]]
    (junction 58) -> AEB_initial_state
    AEB_activation_state -> (junction 58) : [Stop==1]
  data: Time_to_collision output; AEB output; Stop input; TTC input; Action input; Type_of_Collision_Warning output; Selected_Type_of_warning input; Input input; Brake input; Braking_force output; Ego_vehicle_speed input; Time_require_to_match_relative_speed input; Object_speed input; ACC output; Deceleration output; Time_require_to_match_the_speed output; Appied_dece input
